simulink library "radia_simulink_library"  (R2026a)
settings: Solver=VariableStepAuto
undefined symbols (not defined in the file or in its folder): radia, radia_adjoint_runner, radia_electromagnet_adjoint_runner, radia_field_study_bus, radia_ih_geometry_revision, radia_material_bus, radia_motor_angle_family, radia_nonlinear_reactor_config, radia_sheet_metal_runner, radia_streamfunction_adjoint_runner, radia_winding_bus
settings Model: Creator=Administrator  LastModifiedBy=Administrator

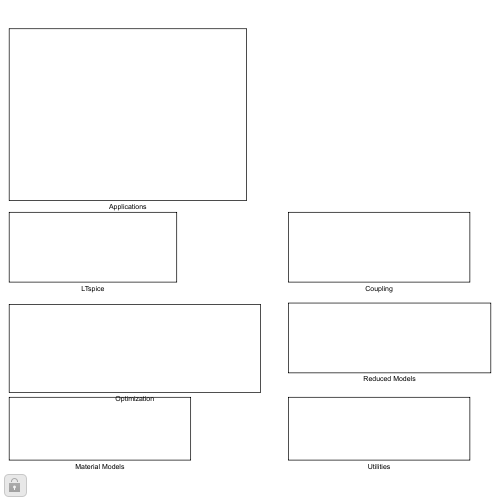
[thumbnail: Simulink's stored preview of the top-level diagram]
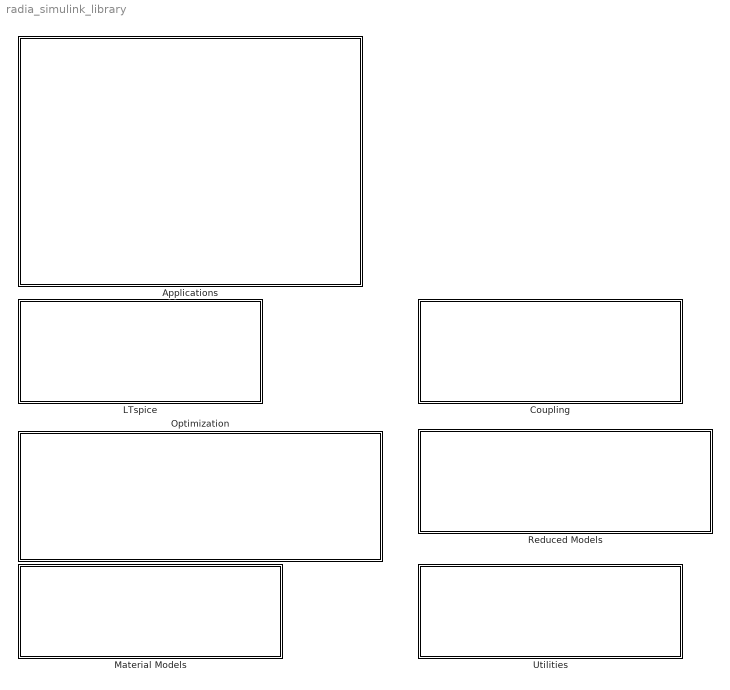
== system radia_simulink_library ==
  Applications : Subsystem
  Coupling : Subsystem
  LTspice : Subsystem
  Material Models : Subsystem
  Optimization : Subsystem
  Reduced Models : Subsystem
  Utilities : Subsystem

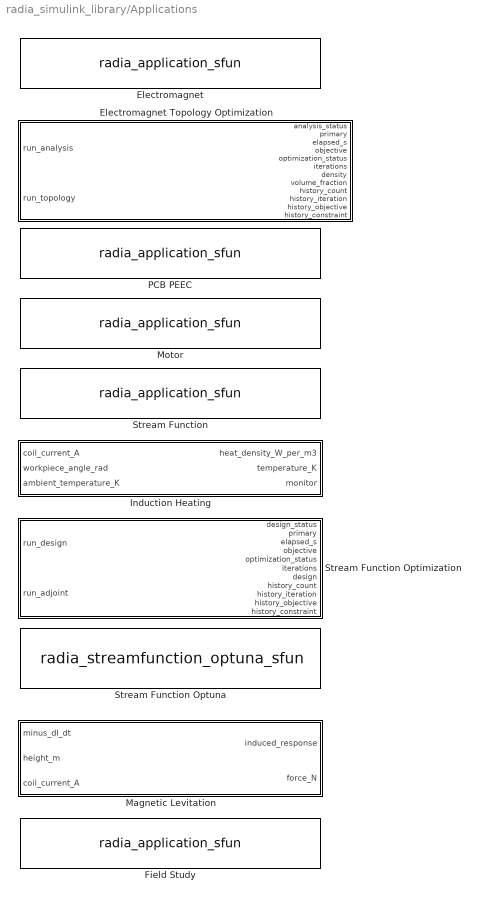
== system radia_simulink_library/Applications ==
  Electromagnet : M-S-Function  FunctionName=radia_application_sfun  Parameters='em', config_file, run_root, timeout_s, python_executable  mask{config_file='', run_root='C:\temp\radia_simulink', timeout_s=3600, python_executable='python'}
      mask prompts: config_file "Configuration JSON"; run_root "Run artifact root"; timeout_s "Timeout (s)"; python_executable "Python executable"
      mask help: Electromagnet batch analysis. Create settings with radia.simulink.writeApplicationConfig; a rising trigger executes the validated Radia headless CLI once.
      mask Display: disp('Electromagnet');port_label('input',1,'run');port_label('output',1,'status');port_label('output',2,'primary');port_label('output',3,'elapsed_s');
  Electromagnet Topology Optimization : Subsystem  Tag=RadiaElectromagnetTopology  mask{config_file='', run_root='C:\temp\radia_simulink', timeout_s=3600, python_executable='python', radia_electromagnet_adjoint_runner=radia_electromagnet_adjoint_runner, solver=mma, sample_time_s=1, history_capacity=96}
      mask prompts: config_file "Analysis configuration JSON"; run_root "Run artifact root"; timeout_s "Timeout (s)"; python_executable "Python executable"; radia_electromagnet_adjoint_runner "Electromagnet adjoint runner"; solver "Optimizer"; sample_time_s "Sample time (s)"; history_capacity "History capacity"
      mask help: Electromagnet batch analysis plus density topology optimization with one VIM state solve, one adjoint solve, and MMA/SQP.
      mask init:
      | radia.simulink.configureElectromagnetOptimizationSubsystem(gcb);
      mask TypeOptions solver: mma | sqp
      mask Display: disp('Electromagnet Topology Optimization');port_label('input',1,'run analysis');port_label('input',2,'run topology');port_label('output',1,'analysis_status');port_label('output',2,'primary');port_label('output',3,'elapsed_s');port_label('output',4,'objective');port_label('output',5,'optimization_status');port_label('output',6,'iterations');port_label('output',7,'density');port_label('output',8,'volume_fraction');port_label('output',9,'history_count');port_label('output',10,'history_iteration');port_label('output',11,'history_objective');port_label('output',12,'history_constraint');
  Field Study : M-S-Function  FunctionName=radia_application_sfun  Parameters='field', config_file, run_root, timeout_s, python_executable  mask{config_file='', run_root='C:\temp\radia_simulink', timeout_s=3600, python_executable='python'}
      mask prompts: config_file "Configuration JSON"; run_root "Run artifact root"; timeout_s "Timeout (s)"; python_executable "Python executable"
      mask help: Field Study batch analysis. Create settings with radia.simulink.writeApplicationConfig; a rising trigger executes the validated Radia headless CLI once.
      mask Display: disp('Field Study');port_label('input',1,'run');port_label('output',1,'status');port_label('output',2,'primary');port_label('output',3,'elapsed_s');
  Induction Heating : Subsystem  mask{config_file=}
      mask prompts: config_file "IHDesignSpec configuration"
      mask help: Native IH preview block. Readable Level-2 MATLAB Eddy and Thermal S-Functions use checked radia_mex handles; raw fields plus an IHMonitorBusV1 output expose physical weighted telemetry.
      mask init:
      | radia.simulink.makeIHMonitorBusObject();
      mask Callback config_file: radia.simulink.onIHConfigFileChanged(gcb);
      mask Display: disp('Induction Heating');port_label('input',1,'I');port_label('input',2,'theta_{work}');port_label('input',3,'T_{amb}');port_label('output',1,'q');port_label('output',2,'T');port_label('output',3,'monitor');
  Magnetic Levitation : Subsystem  Tag=RadiaMagLevFoster  mask{family=radia.simulink.makeMagLevSmokeFamily()}
      mask prompts: family "Shared-mode Foster family"
      mask help: Moving conductive-body HCurl plant in Foster modal form. One mode set is shared by every height; the block evaluates the induced response and reduced Lorentz force without per-step Python.
      mask Callback family: radia.simulink.onMagLevBlockFamilyChanged(gcb);
      mask Display: disp('Magnetic Levitation');port_label('input',1,'-dI/dt');port_label('input',2,'height');port_label('input',3,'I');port_label('output',1,'response');port_label('output',2,'F');
  Motor : M-S-Function  FunctionName=radia_application_sfun  Parameters='motor', config_file, run_root, timeout_s, python_executable  mask{config_file='', run_root='C:\temp\radia_simulink', timeout_s=3600, python_executable='python'}
      mask prompts: config_file "Configuration JSON"; run_root "Run artifact root"; timeout_s "Timeout (s)"; python_executable "Python executable"
      mask help: Motor batch analysis. Create settings with radia.simulink.writeApplicationConfig; a rising trigger executes the validated Radia headless CLI once.
      mask Display: disp('Motor');port_label('input',1,'run');port_label('output',1,'status');port_label('output',2,'primary');port_label('output',3,'elapsed_s');
  PCB PEEC : M-S-Function  FunctionName=radia_application_sfun  Parameters='pcb', config_file, run_root, timeout_s, python_executable  mask{config_file='', run_root='C:\temp\radia_simulink', timeout_s=3600, python_executable='python'}
      mask prompts: config_file "Configuration JSON"; run_root "Run artifact root"; timeout_s "Timeout (s)"; python_executable "Python executable"
      mask help: PCB PEEC batch analysis. Create settings with radia.simulink.writeApplicationConfig; a rising trigger executes the validated Radia headless CLI once.
      mask Display: disp('PCB PEEC');port_label('input',1,'run');port_label('output',1,'status');port_label('output',2,'primary');port_label('output',3,'elapsed_s');
  Stream Function : M-S-Function  FunctionName=radia_application_sfun  Parameters='streamfunction', config_file, run_root, timeout_s, python_executable  mask{config_file='', run_root='C:\temp\radia_simulink', timeout_s=3600, python_executable='python'}
      mask prompts: config_file "Configuration JSON"; run_root "Run artifact root"; timeout_s "Timeout (s)"; python_executable "Python executable"
      mask help: Stream Function batch analysis. Create settings with radia.simulink.writeApplicationConfig; a rising trigger executes the validated Radia headless CLI once.
      mask Display: disp('Stream Function');port_label('input',1,'run');port_label('output',1,'status');port_label('output',2,'primary');port_label('output',3,'elapsed_s');
  Stream Function Optimization : Subsystem  mask{config_file='', run_root='C:\temp\radia_simulink', timeout_s=3600, python_executable='python', radia_streamfunction_adjoint_runner=radia_streamfunction_adjoint_runner, solver=mma, sample_time_s=1, history_capacity=64}
      mask prompts: config_file "Design configuration JSON"; run_root "Run artifact root"; timeout_s "Timeout (s)"; python_executable "Python executable"; radia_streamfunction_adjoint_runner "Stream-function adjoint runner"; solver "Optimizer"; sample_time_s "Sample time (s)"; history_capacity "History capacity"
      mask help: Stream-function design/Pareto batch plus analytic MMA/SQP coefficient optimization and Simulink-native history plots.
      mask init:
      | radia.simulink.configureStreamFunctionOptimizationSubsystem(gcb);
      mask TypeOptions solver: mma | sqp
      mask Display: disp('Stream Function Optimization');port_label('input',1,'run design');port_label('input',2,'run adjoint');port_label('output',1,'design_status');port_label('output',2,'primary');port_label('output',3,'elapsed_s');port_label('output',4,'objective');port_label('output',5,'optimization_status');port_label('output',6,'iterations');port_label('output',7,'design');port_label('output',8,'history_count');port_label('output',9,'history_iteration');port_label('output',10,'history_objective');port_label('output',11,'history_constraint');
  Stream Function Optuna : M-S-Function  FunctionName=radia_streamfunction_optuna_sfun  Parameters=runner_variable,study_variable,num_trials,sample_time_s  mask{runner_variable='radia_streamfunction_optuna_runner', study_variable='radia_streamfunction_optuna_study', num_trials=20, sample_time_s=1}
      mask prompts: runner_variable "Optuna runner variable"; study_variable "Optuna study variable"; num_trials "Number of trials"; sample_time_s "Sample time (s)"
      mask help: MATLAB Optuna outer-loop search over explicit Stream Function ACA+/QR/TSVD batch analyses. One rising trigger runs the requested trials; Python is never called per simulation timestep.
      mask Display: disp('Stream Function Optuna');port_label('input',1,'run');port_label('output',1,'status');port_label('output',2,'best');port_label('output',3,'best trial');port_label('output',4,'completed');port_label('output',5,'failed');port_label('output',6,'pareto N');port_label('output',7,'elapsed_s');

== system radia_simulink_library/Coupling ==
  Field Study Configuration : Subsystem  mask(Radia Field Study){study_contract_variable='radia_field_study_contract', request_file=''}
      mask prompts: study_contract_variable "Field study contract"; request_file "Request JSON"
      mask help: Compile electrostatic, multi-conductor force, current-flow, steady/transient-heat, or linear/nonlinear harmonic-eddy setup to RadiaStudyBus. The Python/NGSolve solve runs once per explicit trigger, not per step.
      mask init:
      | radia.simulink.registerFieldStudy(string(study_contract_variable),RequestFile=string(request_file));
      mask Display: disp('Field Study');port_label('output',1,'study');
  Winding Dictionary : Subsystem  mask(Radia Winding Dictionary){windings_variable='radia_windings', material_contract_variable='radia_material_contract', max_windings=16, max_regions_per_winding=16, max_terminals=32}
      mask prompts: windings_variable "Windings dictionary"; material_contract_variable "Material contract"; max_windings "Maximum windings"; max_regions_per_winding "Maximum regions/winding"; max_terminals "Maximum terminals"
      mask help: Compile winding names, .vol regions, turns, polarity, parallel paths, resistance, and circuit terminals to a fixed-width Bus shared by native MEX and LTspice backends.
      mask init:
      | radia.simulink.registerWindingDictionary(string(windings_variable),string(material_contract_variable),MaxWindings=max_windings,MaxRegionsPerWinding=max_regions_per_winding,MaxTerminals=max_terminals);
      mask Display: disp('Winding Dictionary');port_label('output',1,'windings');

== system radia_simulink_library/LTspice ==
  Hysteretic LTspice Plant : M-S-Function  FunctionName=radia_hysteretic_ltspice_sfun  Parameters='', 1e-3, 'C:\temp\radia_hysteretic_ltspice_block'
  LTspice Circuit : M-S-Function  FunctionName=radia_ltspice_sfun  Parameters='', {'control'}, {'V(out)'}, 1e-3, 'C:\temp\radia_ltspice_block', inf, 300, ''

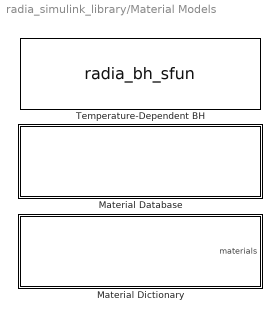
== system radia_simulink_library/Material Models ==
  Material Database : Subsystem  mask{database_file='', material_id='default'}
      mask prompts: database_file "MaterialDatabase MAT/JSON"; material_id "Material ID"
      mask help: Construct and register the immutable workpiece-coordinate MaterialDatabase.
      mask init:
      | if isempty(database_file),error('Material Database requires database_file.');end;[~,~,ext]=fileparts(database_file);if strcmpi(ext,'.mat'),s=load(database_file);if isfield(s,'database'),db=s.database;elseif isfield(s,'radia_material_database'),db=s.radia_material_database;else,error('MAT file must contain database.');end;else,db=jsondecode(fileread(database_file));end;db.material_id=material_id;db=radia.material.validateDatabase(db);assignin('base','radia_material_database',db);
      mask Display: disp('Material Database');
  Material Dictionary : Subsystem  mask(Radia Material Dictionary){materials_variable='radia_materials', region_map_variable='radia_region_materials', mesh_file='', expected_mesh_sha256='', max_materials=32, max_regions=128, max_bh_points=256, max_hysteresis_parameters=16, validate_mesh=on}
      mask prompts: materials_variable "Materials dictionary"; region_map_variable "Region-to-material dictionary"; mesh_file "Netgen .vol mesh"; expected_mesh_sha256 "Expected mesh SHA-256"; max_materials "Maximum materials"; max_regions "Maximum .vol regions"; max_bh_points "Maximum B-H points/material"; max_hysteresis_parameters "Maximum hysteresis parameters/material"; validate_mesh "Run check-vol during initialization"
      mask help: Compile MATLAB material and region dictionaries against a Netgen .vol mesh. The output is a fixed-width numeric Bus for Radia MEX S-Functions; dictionary and string lookup occur only during model initialization.
      mask init:
      | radia.simulink.registerMaterialDictionary(string(materials_variable),string(region_map_variable),string(mesh_file),ExpectedMeshSHA256=string(expected_mesh_sha256),MaxMaterials=max_materials,MaxRegions=max_regions,MaxBHPoints=max_bh_points,MaxHysteresisParameters=max_hysteresis_parameters,ValidateMesh=strcmp(validate_mesh,'on'));
      mask Display: disp('Material Dictionary');port_label('output',1,'materials');
  Temperature-Dependent BH : M-S-Function  FunctionName=radia_bh_sfun  Parameters=radia_bh_config  mask{mode='formula', config_file=''}
      mask prompts: mode "BH mode"; config_file "BH configuration"
      mask help: Temperature-dependent BH law. Select formula or LUT in radia_bh_config.
      mask init:
      | cfg=evalin('base','radia_bh_config');if ~isempty(config_file),s=load(config_file);if isfield(s,'config'),cfg=s.config;elseif isfield(s,'radia_bh_config'),cfg=s.radia_bh_config;else,error('BH config file must contain config or radia_bh_config.');end;end;cfg.mode=mode;assignin('base','radia_bh_config',cfg);
      mask Display: disp('Temperature-Dependent BH');port_label('input',1,'T');port_label('input',2,'H');port_label('output',1,'B');port_label('output',2,'dB/dH');

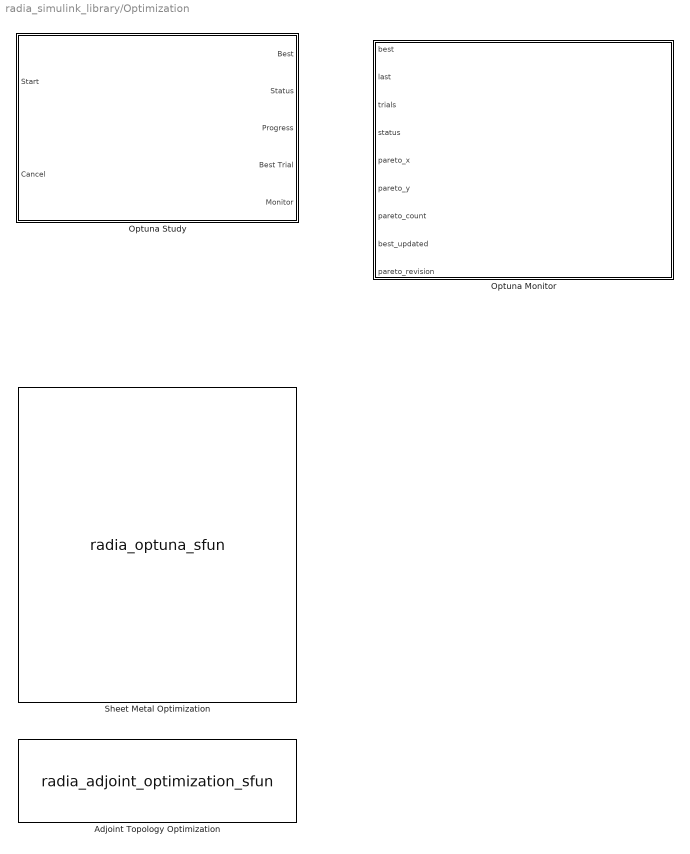
== system radia_simulink_library/Optimization ==
  Adjoint Topology Optimization : M-S-Function  FunctionName=radia_adjoint_optimization_sfun  Parameters=runner,sample_time_s  mask{runner=radia_adjoint_runner, solver=mma, sample_time_s=1}
      mask prompts: runner "AdjointRunner"; solver "Optimizer"; sample_time_s "Sample time (s)"
      mask help: Checked adjoint topology optimization through the MMA/SQP runner.
      mask TypeOptions solver: mma | sqp
      mask Callback solver: runner.setSolver(string(solver));
      mask Display: disp('Adjoint Topology Optimization');port_label('input',1,'start');port_label('output',1,'objective');port_label('output',2,'status');port_label('output',3,'iterations');port_label('output',4,'design');
  Optuna Monitor : Subsystem
      mask help: Simulink-native Optuna history, best-update, and Pareto-front monitor. No browser is used.
      mask Display: disp('Optuna Monitor');port_label('input',1,'best');port_label('input',2,'last');port_label('input',3,'trials');port_label('input',4,'status');port_label('input',5,'pareto_x');port_label('input',6,'pareto_y');port_label('input',7,'pareto_count');port_label('input',8,'best_updated');port_label('input',9,'pareto_revision');
  Optuna Study : Subsystem  mask{objective_fcn='', num_trials=20, directions="minimize", storage_path='', sample_time_s=1, live_visualization=off, sampler_name=auto, seed=[], pruner_name=none, parameter_spec=[], model_name='', selected_trial=-1}
      mask prompts: objective_fcn "Objective function"; num_trials "Total trial budget"; directions "Objective directions"; storage_path "Study MAT file"; sample_time_s "Trial sample time (s)"; live_visualization "External MATLAB monitor"; sampler_name "Sampler"; seed "Sampler seed ([] = fresh)"; pruner_name "Pruner"; parameter_spec "OptimizationParameter array"; model_name "Model to update"; selected_trial "Trial to apply (-1 = best)"
      mask help: Compact MATLAB-native Optuna study. Change the sampler, seed, pruner, search space, or total trial budget in this dialog and run again; the MAT study resumes without changing wiring. OptunaMonitorBusV1 exposes fixed scalar telemetry.
      mask init:
      | radia.simulink.makeOptunaMonitorBusObject();set_param([gcb '/Advanced Runtime'],'Parameters','objective_fcn,num_trials,directions,storage_path,sample_time_s,strcmp(live_visualization,''on''),struct(''Name'',sampler_name,''Seed'',seed,''Pruner'',pruner_name,''Parameters'',parameter_spec,''ModelName'',model_name)');
      mask TypeOptions sampler_name: auto | random | tpe | cmaes | nsgaii | nsgaiii | bruteforce
      mask TypeOptions pruner_name: none | median | hyperband | percentile | patient | successivehalving | threshold
      mask DialogControl review_study Prompt: Review saved study
      mask DialogControl review_study Callback: radia.simulink.reviewOptunaStudy(gcb);
      mask DialogControl apply_trial Prompt: Apply selected trial
      mask DialogControl apply_trial Callback: radia.simulink.applyOptunaTrial(gcb,selected_trial);
      mask Display: disp('Optuna Study');port_label('input',1,'start');port_label('input',2,'cancel');port_label('output',1,'best');port_label('output',2,'status');port_label('output',3,'progress');port_label('output',4,'best trial');port_label('output',5,'monitor');
  Sheet Metal Optimization : M-S-Function  FunctionName=radia_optuna_sfun  Parameters=@(trial)runner.evaluate(trial),num_trials,directions,storage_path,sample_time_s,strcmp(live_visualization,'on'),struct('Name',sampler_name,'Seed',seed,'Pruner',pruner_name,'Parameters',parameter_spec,'ModelName',model_name)  mask{runner=radia_sheet_metal_runner, num_trials=20, directions='minimize', storage_path='', sample_time_s=1, live_visualization=off, sampler_name=auto, seed=[], pruner_name=none, parameter_spec=[], model_name=''}
      mask prompts: runner "SheetMetalRunner"; num_trials "Number of trials"; directions "Objective directions"; storage_path "Study MAT file"; sample_time_s "Trial sample time (s)"; live_visualization "External MATLAB monitor"; sampler_name "Sampler"; seed "Sampler seed ([] = fresh)"; pruner_name "Pruner"; parameter_spec "OptimizationParameter array ([] = Trial objective)"; model_name "Model to update"
      mask help: Native NGSolve/Cubit sheet-metal optimization through radia.optuna.SheetMetalRunner.
      mask TypeOptions sampler_name: auto | random | tpe | cmaes | nsgaii | gp | nsgaiii | bruteforce | qmc
      mask TypeOptions pruner_name: none | median | hyperband | percentile | patient | successivehalving | threshold
      mask Display: disp('Sheet Metal Optimization');port_label('input',1,'start');port_label('input',2,'cancel');port_label('input',3,'pause');port_label('input',4,'resume');port_label('input',5,'selected trial');port_label('input',6,'apply');port_label('output',1,'best');port_label('output',2,'best trial');port_label('output',3,'status');port_label('output',4,'trials');port_label('output',5,'last');port_label('output',6,'elapsed');port_label('output',7,'best update');port_label('output',8,'pareto N');port_label('output',9,'pareto X');port_label('output',10,'pareto Y');port_label('output',11,'pareto rev');port_label('output',12,'failed');port_label('output',13,'attempted');port_label('output',14,'failure code');port_label('output',15,'selected');port_label('output',16,'pruned');port_label('output',17,'current');port_label('output',18,'checkpoint');

== system radia_simulink_library/Reduced Models ==
  Motor Angle Family : M-S-Function  FunctionName=radia_motor_angle_family_mex_sfunction  Parameters=family  mask{family=radia_motor_angle_family}
      mask prompts: family "Motor angle family"
      mask help: Periodic motor ROM with native MEX interpolation, state update, and torque evaluation.
      mask Display: disp('Motor Angle Family');port_label('input',1,'theta,u');port_label('output',1,'y,torque');
  Nonlinear HDiv-MMM Reactor : M-S-Function  FunctionName=radia_nonlinear_reactor_sfun  Parameters=reactor_config  mask(Radia Nonlinear HDiv-MMM Reactor){reactor_config=radia_nonlinear_reactor_config}
      mask prompts: reactor_config "Reactor configuration"
      mask help: Native nonlinear HDiv-MMM reactor. Input is winding current; outputs are terminal voltage, flux linkage, differential inductance, peak B, magnetic energy, Newton iterations, residual, and distributed B samples.
      mask Display: disp('Nonlinear HDiv-MMM Reactor');port_label('input',1,'current_A');port_label('output',1,'voltage_V');port_label('output',2,'flux_Wb_turn');port_label('output',3,'Ldiff_H');port_label('output',4,'Bpeak_T');port_label('output',5,'energy_J');port_label('output',6,'iterations');port_label('output',7,'residual');port_label('output',8,'B_samples_T');

== system radia_simulink_library/Utilities ==
  Field Stats : Subsystem  Tag=RadiaFieldStats
      mask help: Reduces an N-wide field vector (temperature, heat density) to the 3-wide [min mean max] signal for scopes and logging. Base Simulink blocks only; the mean is the arithmetic mean over DOFs (display aid -- volume-weighted means stay owned by the result artifacts).
      mask Display: disp('[min mean max]');

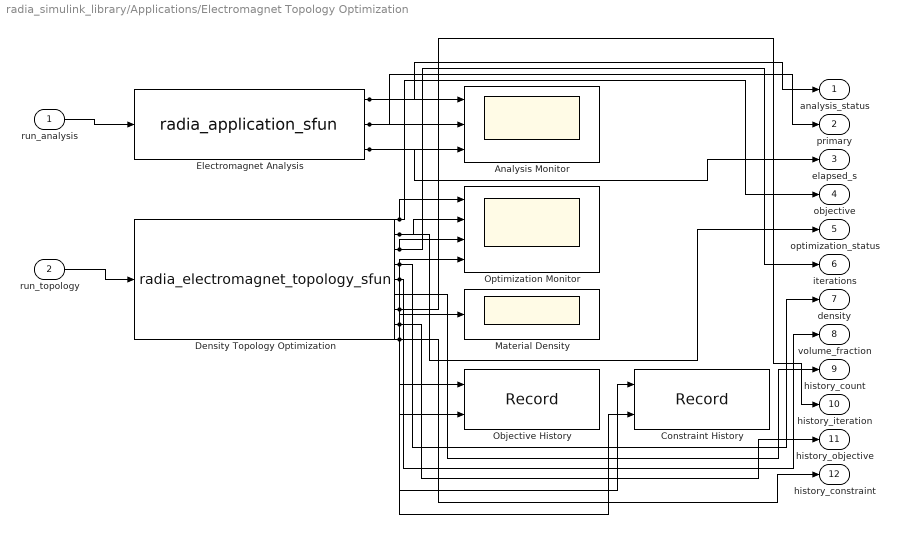
== system radia_simulink_library/Applications/Electromagnet Topology Optimization ==
  run_analysis : Inport  OutDataTypeStr=boolean
  run_topology : Inport  Port=2  OutDataTypeStr=boolean
  Analysis Monitor : Scope  NumInputPorts=3
  Constraint History : Record  NumPorts=2.0  FileSettingsInternal="{\"entries\":[{\"content\":{\"excelSettings\":{\"content\":{},\"type\":\"Streamout.ExcelSettings\"},\"parquetSettings\":{\"content\":{},\"type\":\"Streamout.ParquetSettings\"}},\"type\":\"Streamout.FileSettingStorage\",\"uuid\":\"\"}],\"packageUris\":[\"http:\\/\\/schema.mathworks.com\\/mf0\\/streamout_blocks\\/R2020a\"],\"version\":\"1.0\"}"  FrameSettings=[0, 0]  Layout=[1 1]  SignalsInternal="{\"entries\":[{\"content\":{\"signals\":[{\"content\":{\"blockPath\":[],\"dimensions\":[1],\"domain\":\"\",\"lineColor\":\"#a2142f\",\"plots\":[ 1 ],\"port\":1,\"signalID\":1,\"signalName\":\"XY Graph:1\"},\"type\":\"RecordBlkView.Signal\",\"uuid\":\"\"},{\"content\":{\"blockPath\":[],\"dimensions\":[1],\"domain\":\"\",\"lineColor\":\"#139fff\",\"plots\":[ 1 ],\"port\":2,\"signalID\":2,\"signalName\":\"XY Graph:2\"},\"type\":\"RecordBlkView.Signal\",\"uuid\":\"\"}]},\"type\":\"RecordBlkView.InputSignals\",\"uuid\":\"\"}],\"packageUris\":[\"http:\\/\\/schema.mathworks.com\\/mf0\\/streamout_blocks\\/R2020a\"],\"version\":\"1.0\"}"  VisualizationBindings="{\"xyplotplugin\":{\"info\":[{\"series\":[{\"bindingParametersList\":[{\"parameter\":\"X-Axis\",\"signalID\":1,\"signalName\":\"XY Graph:1\"},{\"parameter\":\"Y-Axis\",\"signalID\":2,\"signalName\":\"XY Graph:2\"}],\"seriesID\":0}],\"subplotID\":1}]}}"  CompatibilityTag=XY
  Density Topology Optimization : M-S-Function  FunctionName=radia_electromagnet_topology_sfun  Parameters=radia_electromagnet_adjoint_runner,1,96
  Electromagnet Analysis : M-S-Function  FunctionName=radia_application_sfun  Parameters='em','','C:\temp\radia_simulink',3600,'python'
  Material Density : Scope
  Objective History : Record  NumPorts=2.0  FileSettingsInternal="{\"entries\":[{\"content\":{\"excelSettings\":{\"content\":{},\"type\":\"Streamout.ExcelSettings\"},\"parquetSettings\":{\"content\":{},\"type\":\"Streamout.ParquetSettings\"}},\"type\":\"Streamout.FileSettingStorage\",\"uuid\":\"\"}],\"packageUris\":[\"http:\\/\\/schema.mathworks.com\\/mf0\\/streamout_blocks\\/R2020a\"],\"version\":\"1.0\"}"  FrameSettings=[0, 0]  Layout=[1 1]  SignalsInternal="{\"entries\":[{\"content\":{\"signals\":[{\"content\":{\"blockPath\":[],\"dimensions\":[1],\"domain\":\"\",\"lineColor\":\"#a2142f\",\"plots\":[ 1 ],\"port\":1,\"signalID\":1,\"signalName\":\"XY Graph:1\"},\"type\":\"RecordBlkView.Signal\",\"uuid\":\"\"},{\"content\":{\"blockPath\":[],\"dimensions\":[1],\"domain\":\"\",\"lineColor\":\"#139fff\",\"plots\":[ 1 ],\"port\":2,\"signalID\":2,\"signalName\":\"XY Graph:2\"},\"type\":\"RecordBlkView.Signal\",\"uuid\":\"\"}]},\"type\":\"RecordBlkView.InputSignals\",\"uuid\":\"\"}],\"packageUris\":[\"http:\\/\\/schema.mathworks.com\\/mf0\\/streamout_blocks\\/R2020a\"],\"version\":\"1.0\"}"  VisualizationBindings="{\"xyplotplugin\":{\"info\":[{\"series\":[{\"bindingParametersList\":[{\"parameter\":\"X-Axis\",\"signalID\":1,\"signalName\":\"XY Graph:1\"},{\"parameter\":\"Y-Axis\",\"signalID\":2,\"signalName\":\"XY Graph:2\"}],\"seriesID\":0}],\"subplotID\":1}]}}"  CompatibilityTag=XY
  Optimization Monitor : Scope  NumInputPorts=4
  analysis_status : Outport
  primary : Outport  Port=2
  elapsed_s : Outport  Port=3
  objective : Outport  Port=4
  optimization_status : Outport  Port=5
  iterations : Outport  Port=6
  density : Outport  Port=7
  volume_fraction : Outport  Port=8
  history_count : Outport  Port=9
  history_iteration : Outport  Port=10
  history_objective : Outport  Port=11
  history_constraint : Outport  Port=12
  wires:
  run_analysis/1 -> Electromagnet Analysis/1
  run_topology/1 -> Density Topology Optimization/1
  Electromagnet Analysis/1 -> analysis_status/1, Analysis Monitor/1
  Electromagnet Analysis/2 -> primary/1, Analysis Monitor/2
  Electromagnet Analysis/3 -> elapsed_s/1, Analysis Monitor/3
  Density Topology Optimization/1 -> objective/1, Optimization Monitor/1
  Density Topology Optimization/2 -> optimization_status/1, Optimization Monitor/2
  Density Topology Optimization/3 -> iterations/1, Optimization Monitor/3
  Density Topology Optimization/4 -> density/1, Material Density/1
  Density Topology Optimization/5 -> volume_fraction/1, Optimization Monitor/4
  Density Topology Optimization/6 -> history_count/1
  Density Topology Optimization/7 -> history_iteration/1, Objective History/1, Constraint History/1
  Density Topology Optimization/8 -> history_objective/1, Objective History/2
  Density Topology Optimization/9 -> history_constraint/1, Constraint History/2

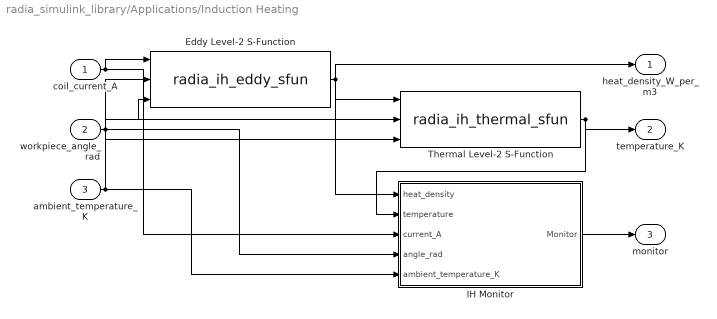
== system radia_simulink_library/Applications/Induction Heating ==
  coil_current_A : Inport
  workpiece_angle_rad : Inport  Port=2
  ambient_temperature_K : Inport  Port=3
  Eddy Level-2 S-Function : M-S-Function  FunctionName=radia_ih_eddy_sfun  Parameters=radia_ih_config
  IH Monitor : Subsystem
      mask help: Native IH scalar telemetry. Internal signal reduction and Bus construction stay encapsulated; raw q and T remain separate.
      mask Display: disp('IH Monitor');port_label('input',1,'q');port_label('input',2,'T');port_label('input',3,'I');port_label('input',4,'theta');port_label('input',5,'T_{amb}');port_label('output',1,'monitor');
  Thermal Level-2 S-Function : M-S-Function  FunctionName=radia_ih_thermal_sfun  Parameters=radia_ih_config
  heat_density_W_per_m3 : Outport
  temperature_K : Outport  Port=2
  monitor : Outport  Port=3
  wires:
  coil_current_A/1 -> Eddy Level-2 S-Function/1, IH Monitor/3(current_A)
  workpiece_angle_rad/1 -> Eddy Level-2 S-Function/2, Thermal Level-2 S-Function/3, IH Monitor/4(angle_rad)
  ambient_temperature_K/1 -> Thermal Level-2 S-Function/2, IH Monitor/5(ambient_temperature_K)
  Eddy Level-2 S-Function/1 -> heat_density_W_per_m3/1, Thermal Level-2 S-Function/1, IH Monitor/1(heat_density)
  Thermal Level-2 S-Function/1 -> temperature_K/1, Eddy Level-2 S-Function/3, IH Monitor/2(temperature)
  IH Monitor/1(Monitor) -> monitor/1

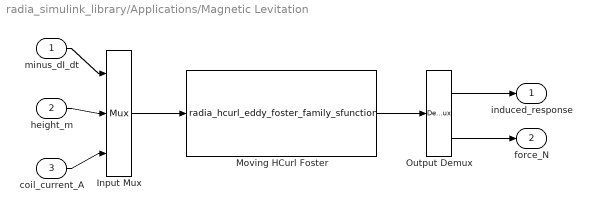
== system radia_simulink_library/Applications/Magnetic Levitation ==
  minus_dI_dt : Inport
  height_m : Inport  Port=2
  coil_current_A : Inport  Port=3
  Input Mux : Mux  Inputs=3
  Moving HCurl Foster : M-S-Function  FunctionName=radia_hcurl_eddy_foster_family_sfunction  Parameters=radia.simulink.makeMagLevSmokeFamily()
  Output Demux : Demux  Outputs=[-1 3]
  induced_response : Outport
  force_N : Outport  Port=2
  wires:
  minus_dI_dt/1 -> Input Mux/1
  height_m/1 -> Input Mux/2
  coil_current_A/1 -> Input Mux/3
  Input Mux/1 -> Moving HCurl Foster/1
  Moving HCurl Foster/1 -> Output Demux/1
  Output Demux/1 -> induced_response/1
  Output Demux/2 -> force_N/1

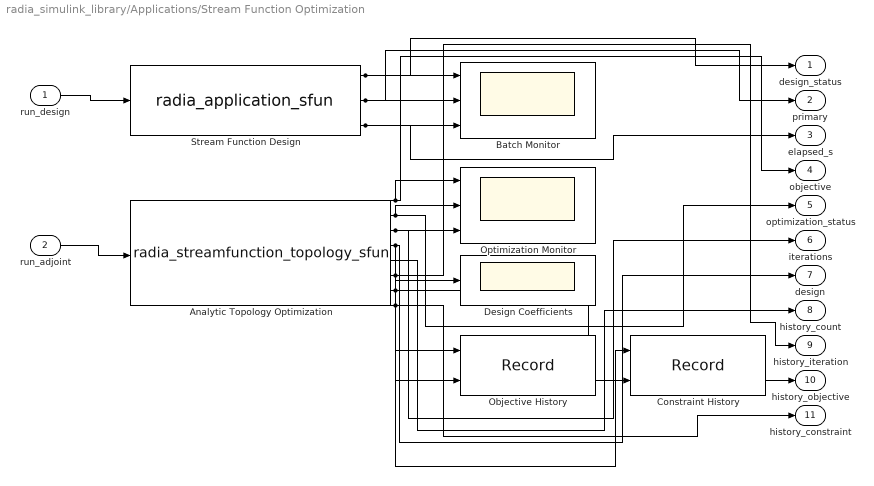
== system radia_simulink_library/Applications/Stream Function Optimization ==
  run_design : Inport  OutDataTypeStr=boolean
  run_adjoint : Inport  Port=2  OutDataTypeStr=boolean
  Analytic Topology Optimization : M-S-Function  FunctionName=radia_streamfunction_topology_sfun  Parameters=radia_streamfunction_adjoint_runner,1,64
  Batch Monitor : Scope  NumInputPorts=3
  Constraint History : Record  NumPorts=2.0  FileSettingsInternal="{\"entries\":[{\"content\":{\"excelSettings\":{\"content\":{},\"type\":\"Streamout.ExcelSettings\"},\"parquetSettings\":{\"content\":{},\"type\":\"Streamout.ParquetSettings\"}},\"type\":\"Streamout.FileSettingStorage\",\"uuid\":\"\"}],\"packageUris\":[\"http:\\/\\/schema.mathworks.com\\/mf0\\/streamout_blocks\\/R2020a\"],\"version\":\"1.0\"}"  FrameSettings=[0, 0]  Layout=[1 1]  SignalsInternal="{\"entries\":[{\"content\":{\"signals\":[{\"content\":{\"blockPath\":[],\"dimensions\":[1],\"domain\":\"\",\"lineColor\":\"#a2142f\",\"plots\":[ 1 ],\"port\":1,\"signalID\":1,\"signalName\":\"XY Graph:1\"},\"type\":\"RecordBlkView.Signal\",\"uuid\":\"\"},{\"content\":{\"blockPath\":[],\"dimensions\":[1],\"domain\":\"\",\"lineColor\":\"#139fff\",\"plots\":[ 1 ],\"port\":2,\"signalID\":2,\"signalName\":\"XY Graph:2\"},\"type\":\"RecordBlkView.Signal\",\"uuid\":\"\"}]},\"type\":\"RecordBlkView.InputSignals\",\"uuid\":\"\"}],\"packageUris\":[\"http:\\/\\/schema.mathworks.com\\/mf0\\/streamout_blocks\\/R2020a\"],\"version\":\"1.0\"}"  VisualizationBindings="{\"xyplotplugin\":{\"info\":[{\"series\":[{\"bindingParametersList\":[{\"parameter\":\"X-Axis\",\"signalID\":1,\"signalName\":\"XY Graph:1\"},{\"parameter\":\"Y-Axis\",\"signalID\":2,\"signalName\":\"XY Graph:2\"}],\"seriesID\":0}],\"subplotID\":1}]}}"  CompatibilityTag=XY
  Design Coefficients : Scope
  Objective History : Record  NumPorts=2.0  FileSettingsInternal="{\"entries\":[{\"content\":{\"excelSettings\":{\"content\":{},\"type\":\"Streamout.ExcelSettings\"},\"parquetSettings\":{\"content\":{},\"type\":\"Streamout.ParquetSettings\"}},\"type\":\"Streamout.FileSettingStorage\",\"uuid\":\"\"}],\"packageUris\":[\"http:\\/\\/schema.mathworks.com\\/mf0\\/streamout_blocks\\/R2020a\"],\"version\":\"1.0\"}"  FrameSettings=[0, 0]  Layout=[1 1]  SignalsInternal="{\"entries\":[{\"content\":{\"signals\":[{\"content\":{\"blockPath\":[],\"dimensions\":[1],\"domain\":\"\",\"lineColor\":\"#a2142f\",\"plots\":[ 1 ],\"port\":1,\"signalID\":1,\"signalName\":\"XY Graph:1\"},\"type\":\"RecordBlkView.Signal\",\"uuid\":\"\"},{\"content\":{\"blockPath\":[],\"dimensions\":[1],\"domain\":\"\",\"lineColor\":\"#139fff\",\"plots\":[ 1 ],\"port\":2,\"signalID\":2,\"signalName\":\"XY Graph:2\"},\"type\":\"RecordBlkView.Signal\",\"uuid\":\"\"}]},\"type\":\"RecordBlkView.InputSignals\",\"uuid\":\"\"}],\"packageUris\":[\"http:\\/\\/schema.mathworks.com\\/mf0\\/streamout_blocks\\/R2020a\"],\"version\":\"1.0\"}"  VisualizationBindings="{\"xyplotplugin\":{\"info\":[{\"series\":[{\"bindingParametersList\":[{\"parameter\":\"X-Axis\",\"signalID\":1,\"signalName\":\"XY Graph:1\"},{\"parameter\":\"Y-Axis\",\"signalID\":2,\"signalName\":\"XY Graph:2\"}],\"seriesID\":0}],\"subplotID\":1}]}}"  CompatibilityTag=XY
  Optimization Monitor : Scope  NumInputPorts=3
  Stream Function Design : M-S-Function  FunctionName=radia_application_sfun  Parameters='streamfunction','','C:\temp\radia_simulink',3600,'python'
  design_status : Outport
  primary : Outport  Port=2
  elapsed_s : Outport  Port=3
  objective : Outport  Port=4
  optimization_status : Outport  Port=5
  iterations : Outport  Port=6
  design : Outport  Port=7
  history_count : Outport  Port=8
  history_iteration : Outport  Port=9
  history_objective : Outport  Port=10
  history_constraint : Outport  Port=11
  wires:
  run_design/1 -> Stream Function Design/1
  run_adjoint/1 -> Analytic Topology Optimization/1
  Stream Function Design/1 -> design_status/1, Batch Monitor/1
  Stream Function Design/2 -> primary/1, Batch Monitor/2
  Stream Function Design/3 -> elapsed_s/1, Batch Monitor/3
  Analytic Topology Optimization/1 -> objective/1, Optimization Monitor/1
  Analytic Topology Optimization/2 -> optimization_status/1, Optimization Monitor/2
  Analytic Topology Optimization/3 -> iterations/1, Optimization Monitor/3
  Analytic Topology Optimization/4 -> design/1, Design Coefficients/1
  Analytic Topology Optimization/5 -> history_count/1
  Analytic Topology Optimization/6 -> history_iteration/1, Objective History/1, Constraint History/1
  Analytic Topology Optimization/7 -> history_objective/1, Objective History/2
  Analytic Topology Optimization/8 -> history_constraint/1, Constraint History/2

== system radia_simulink_library/Coupling/Field Study Configuration ==
  Compiled Study Bus : Constant  Value=radia_field_study_bus  OutDataTypeStr=Bus: RadiaStudyBus
  study : Outport
  wires:
  Compiled Study Bus/1 -> study/1

== system radia_simulink_library/Coupling/Winding Dictionary ==
  Compiled Winding Bus : Constant  Value=radia_winding_bus  OutDataTypeStr=Bus: RadiaWindingBus
  windings : Outport
  wires:
  Compiled Winding Bus/1 -> windings/1

== system radia_simulink_library/Material Models/Material Database ==

== system radia_simulink_library/Material Models/Material Dictionary ==
  Compiled Material Bus : Constant  Value=radia_material_bus  OutDataTypeStr=Bus: RadiaMaterialBus
  materials : Outport
  wires:
  Compiled Material Bus/1 -> materials/1

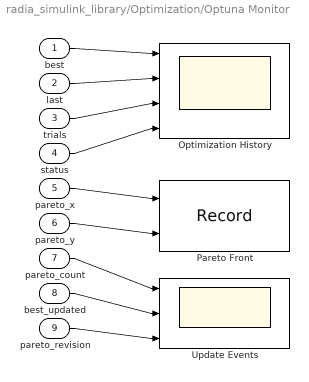
== system radia_simulink_library/Optimization/Optuna Monitor ==
  best : Inport
  last : Inport  Port=2
  trials : Inport  Port=3
  status : Inport  Port=4
  pareto_x : Inport  Port=5
  pareto_y : Inport  Port=6
  pareto_count : Inport  Port=7
  best_updated : Inport  Port=8
  pareto_revision : Inport  Port=9
  Optimization History : Scope  NumInputPorts=4
  Pareto Front : Record  NumPorts=2.0  FileSettingsInternal="{\"entries\":[{\"content\":{\"excelSettings\":{\"content\":{},\"type\":\"Streamout.ExcelSettings\"},\"parquetSettings\":{\"content\":{},\"type\":\"Streamout.ParquetSettings\"}},\"type\":\"Streamout.FileSettingStorage\",\"uuid\":\"\"}],\"packageUris\":[\"http:\\/\\/schema.mathworks.com\\/mf0\\/streamout_blocks\\/R2020a\"],\"version\":\"1.0\"}"  FrameSettings=[0, 0]  Layout=[1 1]  SignalsInternal="{\"entries\":[{\"content\":{\"signals\":[{\"content\":{\"blockPath\":[],\"dimensions\":[1],\"domain\":\"\",\"lineColor\":\"#a2142f\",\"plots\":[ 1 ],\"port\":1,\"signalID\":1,\"signalName\":\"XY Graph:1\"},\"type\":\"RecordBlkView.Signal\",\"uuid\":\"\"},{\"content\":{\"blockPath\":[],\"dimensions\":[1],\"domain\":\"\",\"lineColor\":\"#139fff\",\"plots\":[ 1 ],\"port\":2,\"signalID\":2,\"signalName\":\"XY Graph:2\"},\"type\":\"RecordBlkView.Signal\",\"uuid\":\"\"}]},\"type\":\"RecordBlkView.InputSignals\",\"uuid\":\"\"}],\"packageUris\":[\"http:\\/\\/schema.mathworks.com\\/mf0\\/streamout_blocks\\/R2020a\"],\"version\":\"1.0\"}"  VisualizationBindings="{\"xyplotplugin\":{\"info\":[{\"series\":[{\"bindingParametersList\":[{\"parameter\":\"X-Axis\",\"signalID\":1,\"signalName\":\"XY Graph:1\"},{\"parameter\":\"Y-Axis\",\"signalID\":2,\"signalName\":\"XY Graph:2\"}],\"seriesID\":0}],\"subplotID\":1}]}}"  CompatibilityTag=XY
  Update Events : Scope  NumInputPorts=3
  wires:
  best/1 -> Optimization History/1
  last/1 -> Optimization History/2
  trials/1 -> Optimization History/3
  status/1 -> Optimization History/4
  pareto_x/1 -> Pareto Front/1
  pareto_y/1 -> Pareto Front/2
  pareto_count/1 -> Update Events/1
  best_updated/1 -> Update Events/2
  pareto_revision/1 -> Update Events/3

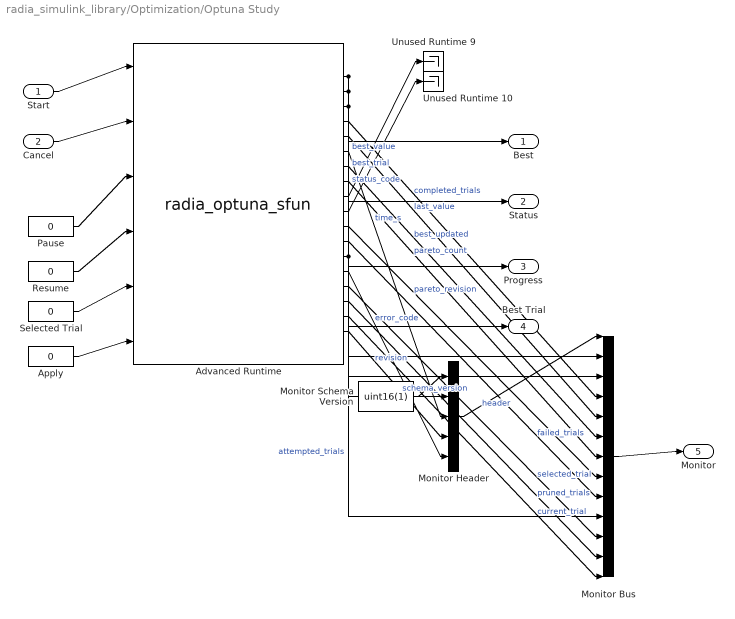
== system radia_simulink_library/Optimization/Optuna Study ==
  Start : Inport
  Cancel : Inport  Port=2
  Advanced Runtime : M-S-Function  FunctionName=radia_optuna_sfun  Parameters="'',20,\"minimize\",'',1,0,struct('Name','auto','Seed',[],'Pruner','none','Parameters',[],'ModelName','')"
  Apply : Constant  Value=0
  Monitor Bus : BusCreator  Inputs=13  OutDataTypeStr=Bus: OptunaMonitorBusV1  NonVirtualBus=on
  Monitor Header : BusCreator  Inputs=5  OutDataTypeStr=Bus: RadiaMonitorHeaderV1  NonVirtualBus=on
  Monitor Schema Version : Constant  Value=uint16(1)  OutDataTypeStr=uint16
  Pause : Constant  Value=0
  Resume : Constant  Value=0
  Selected Trial : Constant  Value=0
  Unused Runtime 10 : Terminator
  Unused Runtime 9 : Terminator
  Best : Outport
  Status : Outport  Port=2
  Progress : Outport  Port=3
  Best Trial : Outport  Port=4
  Monitor : Outport  Port=5
  wires:
  Start/1 -> Advanced Runtime/1
  Cancel/1 -> Advanced Runtime/2
  Pause/1 -> Advanced Runtime/3
  Resume/1 -> Advanced Runtime/4
  Selected Trial/1 -> Advanced Runtime/5
  Apply/1 -> Advanced Runtime/6
  Advanced Runtime/1 -> Best/1, Monitor Bus/2  "best_value"
  Advanced Runtime/3 -> Status/1, Monitor Header/2  "status_code"
  Advanced Runtime/13 -> Progress/1, Monitor Bus/10  "attempted_trials"
  Advanced Runtime/2 -> Best Trial/1, Monitor Bus/3  "best_trial"
  Monitor Schema Version/1 -> Monitor Header/1  "schema_version"
  Advanced Runtime/6 -> Monitor Header/3  "time_s"
  Advanced Runtime/18 -> Monitor Header/4  "revision"
  Advanced Runtime/14 -> Monitor Header/5  "error_code"
  Monitor Header/1 -> Monitor Bus/1  "header"
  Advanced Runtime/4 -> Monitor Bus/4  "completed_trials"
  Advanced Runtime/5 -> Monitor Bus/5  "last_value"
  Advanced Runtime/7 -> Monitor Bus/6  "best_updated"
  Advanced Runtime/8 -> Monitor Bus/7  "pareto_count"
  Advanced Runtime/11 -> Monitor Bus/8  "pareto_revision"
  Advanced Runtime/12 -> Monitor Bus/9  "failed_trials"
  Advanced Runtime/15 -> Monitor Bus/11  "selected_trial"
  Advanced Runtime/16 -> Monitor Bus/12  "pruned_trials"
  Advanced Runtime/17 -> Monitor Bus/13  "current_trial"
  Monitor Bus/1 -> Monitor/1
  Advanced Runtime/9 -> Unused Runtime 9/1
  Advanced Runtime/10 -> Unused Runtime 10/1

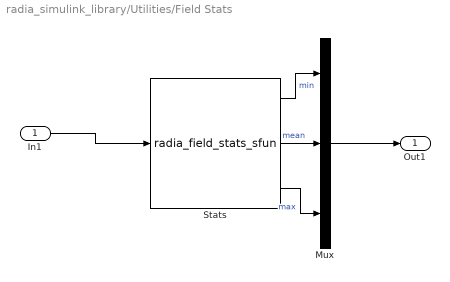
== system radia_simulink_library/Utilities/Field Stats ==
  In1 : Inport
  Mux : Mux  Inputs=3
  Stats : M-S-Function  FunctionName=radia_field_stats_sfun
  Out1 : Outport
  wires:
  In1/1 -> Stats/1
  Stats/1 -> Mux/1  "min"
  Stats/2 -> Mux/2  "mean"
  Stats/3 -> Mux/3  "max"
  Mux/1 -> Out1/1

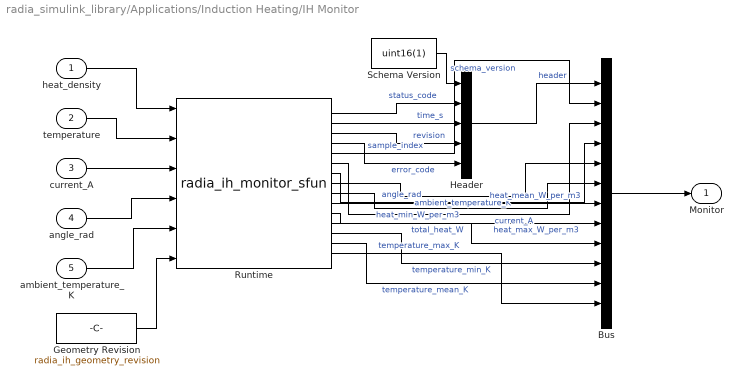
== system radia_simulink_library/Applications/Induction Heating/IH Monitor ==
  heat_density : Inport
  temperature : Inport  Port=2
  current_A : Inport  Port=3
  angle_rad : Inport  Port=4
  ambient_temperature_K : Inport  Port=5
  Bus : BusCreator  Inputs=12  OutDataTypeStr=Bus: IHMonitorBusV1  NonVirtualBus=on
  Geometry Revision : Constant  Value=radia_ih_geometry_revision
  Header : BusCreator  Inputs=5  OutDataTypeStr=Bus: RadiaMonitorHeaderV1  NonVirtualBus=on
  Runtime : M-S-Function  FunctionName=radia_ih_monitor_sfun  Parameters=radia_ih_config
  Schema Version : Constant  Value=uint16(1)  OutDataTypeStr=uint16
  Monitor : Outport
  wires:
  heat_density/1 -> Runtime/1
  temperature/1 -> Runtime/2
  current_A/1 -> Runtime/3
  angle_rad/1 -> Runtime/4
  ambient_temperature_K/1 -> Runtime/5
  Geometry Revision/1 -> Runtime/6
  Schema Version/1 -> Header/1  "schema_version"
  Runtime/1 -> Header/2  "status_code"
  Runtime/2 -> Header/3  "time_s"
  Runtime/3 -> Header/4  "revision"
  Runtime/4 -> Header/5  "error_code"
  Header/1 -> Bus/1  "header"
  Runtime/5 -> Bus/2  "sample_index"
  Runtime/6 -> Bus/3  "current_A"
  Runtime/7 -> Bus/4  "angle_rad"
  Runtime/8 -> Bus/5  "ambient_temperature_K"
  Runtime/9 -> Bus/6  "heat_min_W_per_m3"
  Runtime/10 -> Bus/7  "heat_mean_W_per_m3"
  Runtime/11 -> Bus/8  "heat_max_W_per_m3"
  Runtime/12 -> Bus/9  "total_heat_W"
  Runtime/13 -> Bus/10  "temperature_min_K"
  Runtime/14 -> Bus/11  "temperature_mean_K"
  Runtime/15 -> Bus/12  "temperature_max_K"
  Bus/1 -> Monitor/1
